simulink model "input_display"  (R2015a)
settings: configuration reference "config_cosim" (kept outside this file)
PreLoadFcn:
  | load config_cosim
model workspace (MAT data in the model file):
  Target.Ind = [1 0 1 0 0 0 1 0]
  Target.FSC = [1 0 1 0 0 0 4 0]
  Target.DD = [1  0; 0  0; 0  1; 0  0; 0  0; 0  0; 0  1; 0  0]
  Target.Ind0 = 0
  cmd_asn_cfm1 = [1 0 1 0 0 0 1 0]
  t_delta = 1
settings Model: CovModelRefEnable=off  Creator=zhang  LastModifiedBy=yrzhang
settings ConfigSetRef: SourceLocation=Base Workspace

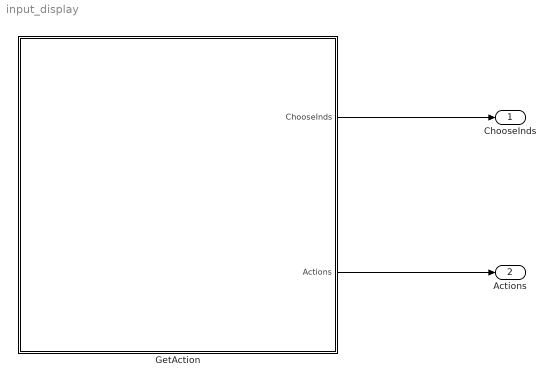
== system input_display ==
  GetAction : Stateflow chart  TreatAsAtomicUnit=on
  ChooseInds : Outport  OutDataTypeStr=Bus: ChooseBusObject
  Actions : Outport  Port=2  OutDataTypeStr=Bus: ActionBusObject
  wires:
  GetAction/2(Actions) -> Actions/1
  GetAction/1(ChooseInds) -> ChooseInds/1

== stateflow chart input_display/GetAction ==
  state GetActionData
    state TgtAsnMode [parallel]
      entry,during: coder.extrinsic('display_control');
      [~,ChooseInds.TgtAsnInd,ChooseInds.MslInd,Actions.TgtAsn,Actions.TgtAsnCcl] = display_control('GetAsnAction');
      settings: executionOrder=1
    state TgtPwrMode [parallel]
      entry,during: coder.extrinsic('display_control');
      [~,ChooseInds.PwrInd,Actions.PwrOn,Actions.PwrOff] = display_control('GetPwrAction');
      settings: executionOrder=2
    state TgtFSMode [parallel]
      entry,during: coder.extrinsic('display_control');
      [~,ChooseInds.TgtFsInd,Actions.FS] = display_control('GetFSAction');
      settings: executionOrder=3
  (default) -> GetActionData : % 初始化用户操作
      | {coder.extrinsic('display_control');
      | Actions.PwrOn = 0;
      | Actions.PwrOff = 1;
      | Actions.FS = 0;Actions.TgtAsn = 0;
      | Actions.TgtAsnCcl = 0;
      | ChooseInds.TgtAsnInd = 0;
      | ChooseInds.MslInd = [0;0];
      | ChooseInds.PwrInd = false(8,1);
      | ChooseInds.TgtFsInd = [0 0;0 0;0 0;0 0;0 0;0 0;0 0;0 0];
      | }
  data: ChooseInds output Bus: ChooseBusObject; Actions output Bus: ActionBusObject
